simulink model "PCM_accurate"  (R2023a)
settings: Solver=VariableStepAuto  StartTime=0.0  StopTime=.008  FixedStep=.00001  MaxStep=.000001  RelTol=1e-3
values from neighbouring files (symbols this model uses):
  C = 10*10^-6    (= 1e-05)    [parameters.m]
  Fs = 75*10^3    (= 75000)    [parameters.m]
  L = 220*10^-6    (= 0.00022)    [parameters.m]
  Ma = M2    (= 54545.4545455)    [parameters.m]
  R = 5    [parameters.m]
  Vin = 48    [parameters.m]
libraries: spsSeriesRLCBranchLib x4, spsCurrentMeasurementLib x3, spsControlledVoltageSourceLib x1, spsDiodeLib x1, spsIdealSwitchLib x1, spsMosfetLib x1, simulink_extras x1, spsVoltageMeasurementLib x1, spspowerguiLib x1
settings Model: Creator=User  LastModifiedBy=User
settings DebuggingCC: IgnoredZcDiagnostic=none  UnconnectedInputMsg=warning  UnconnectedOutputMsg=warning  UnconnectedLineMsg=warning
settings ModelReferenceCC: EnableRefExpFcnMdlSchedulingChecks=on
settings RTWCC: DLArmComputeVersion=19.05

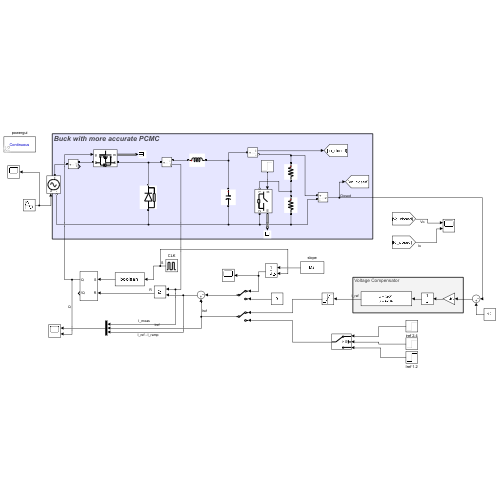
[thumbnail: Simulink's stored preview of the top-level diagram]
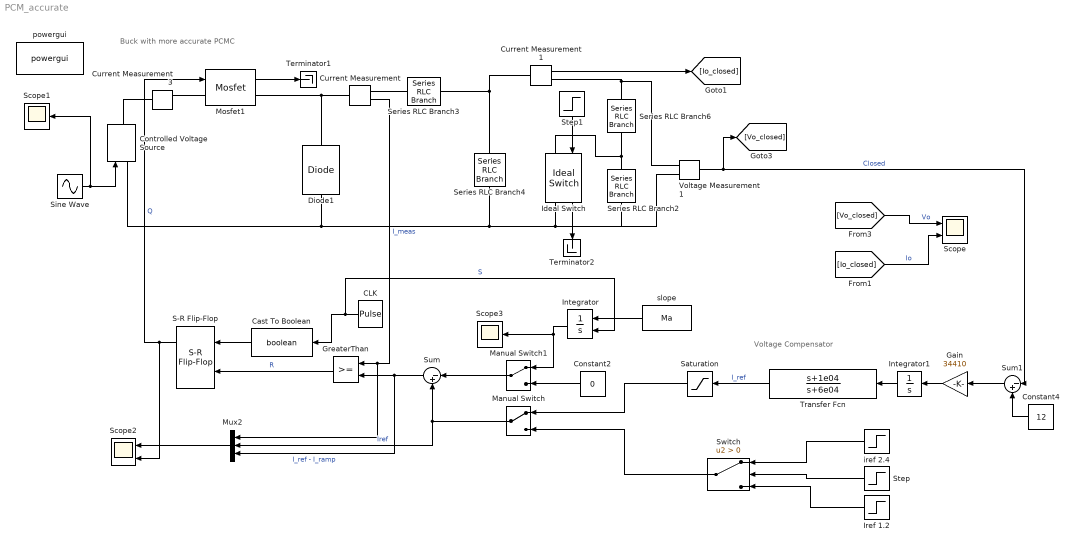
== system PCM_accurate ==
  note: Voltage Compensator
  note: Buck with more accurate PCMC
  CLK : DiscretePulseGenerator  PulseType=Time based  Period=1/Fs  PulseWidth=10
  Cast To Boolean : DataTypeConversion  OutDataTypeStr=boolean  SaturateOnIntegerOverflow=off  RndMeth=Floor
  Constant2 : Constant  Value=0
  Constant4 : Constant  Value=12
  Controlled Voltage Source : spsControlledVoltageSourceLib/Controlled Voltage Source  Initialize=on  Source_Type=AC  Amplitude=0  Phase=0  Frequency=0  Measurements=None
  Current Measurement : spsCurrentMeasurementLib/Current Measurement  PhasorSimulation=off  OutputType=Complex  PSBequivalent=0
  Current Measurement1 : spsCurrentMeasurementLib/Current Measurement  PhasorSimulation=off  OutputType=Complex  PSBequivalent=0
  Current Measurement3 : spsCurrentMeasurementLib/Current Measurement  PhasorSimulation=off  OutputType=Complex  PSBequivalent=0
  Diode1 : spsDiodeLib/Diode  Ron=0.001  Lon=0  Vf=0.8  IC=0  UseSnubber=0  Rs=500  Cs=250e-9  Measurements=off
  Gain : Gain  Gain=34410
  GreaterThan : RelationalOperator  OutDataTypeStr=boolean  RndMeth=Simplest  InputSameDT=off
  Ideal Switch : spsIdealSwitchLib/Ideal Switch  Ron=0.001  Lon=0  IC=0  Rs=1e5  Cs=inf  Measurements=on
  Integrator : Integrator  ExternalReset=rising
  Integrator1 : Integrator
  Iref 1.2 : Step  Time=0  After=1.2  SampleTime=0
  Manual Switch : ManualSwitch
  Manual Switch1 : ManualSwitch
  Mosfet1 : spsMosfetLib/Mosfet  Ron=0.1  Lon=0  Rd=0.01  Vfd=0  IC=0  Rs=1e5  Cs=inf  Measurements=on
  Mux2 : Mux  Inputs=3
  S-R Flip-Flop : simulink_extras/Flip Flops/S-R Flip-Flop  initial_condition=0
  Saturation : Saturate  UpperLimit=inf  LowerLimit=0
  Scope : Scope  NumInputPorts=2
  Scope1 : Scope
  Scope2 : Scope  NumInputPorts=2
  Scope3 : Scope
  Series RLC Branch2 : spsSeriesRLCBranchLib/Series RLC Branch  LConnTagsString=__new0  RConnTagsString=__new0  BranchType=R  Resistance=.5*R  Inductance=1e-3  SetiL0=off  InitialCurrent=0  Capacitance=1e-6  Setx0=off  InitialVoltage=0  Measurements=None
  Series RLC Branch3 : spsSeriesRLCBranchLib/Series RLC Branch  LConnTagsString=__new0  RConnTagsString=__new0  BranchType=L  Resistance=1  Inductance=L  SetiL0=off  InitialCurrent=0  Capacitance=1e-6  Setx0=off  InitialVoltage=0  Measurements=None
  Series RLC Branch4 : spsSeriesRLCBranchLib/Series RLC Branch  LConnTagsString=__new0  RConnTagsString=__new0  BranchType=C  Resistance=1  Inductance=1e-3  SetiL0=off  InitialCurrent=0  Capacitance=C  Setx0=off  InitialVoltage=0  Measurements=None
  Series RLC Branch6 : spsSeriesRLCBranchLib/Series RLC Branch  LConnTagsString=__new0  RConnTagsString=__new0  BranchType=R  Resistance=.5*R  Inductance=1e-3  SetiL0=off  InitialCurrent=0  Capacitance=1e-6  Setx0=off  InitialVoltage=0  Measurements=None
  Sine Wave : Sin  Amplitude=2  Bias=Vin  Frequency=2*pi*100  SampleTime=0
  Step : Step  Time=.15  SampleTime=0
  Step1 : Step  Time=.004  SampleTime=0
  Sum : Sum  Inputs=|-+
  Sum1 : Sum  Inputs=|-+
  Switch : Switch  Criteria=u2 > Threshold  SaturateOnIntegerOverflow=off  InputSameDT=off
  Terminator1 : Terminator
  Terminator2 : Terminator
  Transfer Fcn : TransferFcn  Numerator=[1 1e04]  Denominator=[1 6e04]
  Voltage Measurement1 : spsVoltageMeasurementLib/Voltage Measurement  PhasorSimulation=off  OutputType=Complex  PSBequivalent=0
  iref 2.4 : Step  Time=.15  Before=2.4  After=2.4  SampleTime=0
  powergui : spspowerguiLib/powergui  Priority=1  SimulationMode=Continuous  SampleTime=50e-6  frequency=60  Iterations=50  frequencyindice=0  Pbase=100e6  ErrMax=1e-4  UnitsV=kV  UnitsW=MW  buscounter=0  FunctionMessages=off  echomessages=off  EnableUseOfTLC=off  CurrentSourceSwitches=off  DisableSnubberDevices=off  DisableRonSwitches=off  DisableVfSwitches=off  DisplayEquations=off  AutomaticDiscreteSolvers=off  SolverType=Tustin/Backward Euler (TBE)  Interpol=off  ExternalGateDelay=off  methode=off  Ts=100  x0status=blocks  SPID=on  SwTol=0  HookPort=off  NonlinearTolerance=1e-4  nMaxIteration=100  ContinueOnMaxIteration=off  RestoreLinks=warning  ResistiveCurrentMeasurement=off  Frange=[0:2:500]  Ylog=off  Xlog=on  ShowGrid=off  save=off  variable=ZData  structure=0  ZoomFFT=off  StartTime=0.0  cycles=1  DisplayStyle=1  fundamental=60  FreqAxis=off  MaxFrequency=1000  frequencyindicesteady=1  RmsSteady=1  display=off
  slope : Constant  Value=Ma
  wires:
  Mosfet1/1 -> Terminator1/1
  Voltage Measurement1/1 -> [Vo_closed], Sum1/1  "Closed"
  Sum1/1 -> Gain/1
  Transfer Fcn/1 -> Saturation/1  "I_ref"
  S-R Flip-Flop/1 -> Scope2/2, Mosfet1/1  "Q"
  Integrator1/1 -> Transfer Fcn/1
  Current Measurement1/1 -> [Io_closed]
  [Io_closed] -> Scope/2  "Io"
  [Vo_closed] -> Scope/1  "Vo"
  Constant4/1 -> Sum1/2
  Sine Wave/1 -> Scope1/1, Controlled Voltage Source/1
  Current Measurement/1 -> Mux2/1, GreaterThan/1  "I_meas"
  GreaterThan/1 -> S-R Flip-Flop/2  "R"
  CLK/1 -> Cast To Boolean/1, Integrator/2  "S"
  Cast To Boolean/1 -> S-R Flip-Flop/1
  Saturation/1 -> Manual Switch/1
  Iref 1.2/1 -> Switch/3
  Manual Switch/1 -> Sum/2, Mux2/2  "Iref"
  Mux2/1 -> Scope2/1
  iref 2.4/1 -> Switch/1
  Step/1 -> Switch/2
  Switch/1 -> Manual Switch/2
  Sum/1 -> Mux2/3, GreaterThan/2  "I_ref - I_ramp"
  slope/1 -> Integrator/1
  Integrator/1 -> Scope3/1, Manual Switch1/1
  Constant2/1 -> Manual Switch1/2
  Manual Switch1/1 -> Sum/1
  Gain/1 -> Integrator1/1
  Ideal Switch/1 -> Terminator2/1
  Step1/1 -> Ideal Switch/1
  connections:
  Ideal Switch/RConn1 -- Series RLC Branch2/RConn1 -- Voltage Measurement1/LConn2 -- Series RLC Branch4/RConn1 -- Diode1/LConn1 -- Controlled Voltage Source/LConn1
  Diode1/RConn1 -- Mosfet1/RConn1 -- Current Measurement/LConn1
  Current Measurement3/LConn1 -- Controlled Voltage Source/RConn1
  Series RLC Branch4/LConn1 -- Series RLC Branch3/RConn1 -- Current Measurement1/LConn1
  Mosfet1/LConn1 -- Current Measurement3/RConn1
  Voltage Measurement1/LConn1 -- Current Measurement1/RConn1 -- Series RLC Branch6/LConn1
  Current Measurement/RConn1 -- Series RLC Branch3/LConn1
  Series RLC Branch6/RConn1 -- Ideal Switch/LConn1 -- Series RLC Branch2/LConn1
